simulink model "Model16"  (R2016a)
settings: Solver=FixedStepAuto  StartTime=0  StopTime=inf  FixedStep=0.1  RelTol=1e-3
model workspace (MAT data in the model file):
  c1input = 17
  c2input = 1
  u = 2.9338
settings Model: Creator=CAMILO ANDRES  LastModifiedBy=Luis de la Torre
settings DataIOCC: LimitDataPoints=on  SaveFormat=Array  SaveOutput=off  SignalLogging=off  DSMLogging=off  SaveTime=off
settings DebuggingCC: UnderspecifiedInitializationDetection=Classic  MergeDetectMultiDrivingBlocksExec=none  SolverPrmCheckMsg=warning  FcnCallInpInsideContextMsg=EnableAllAsWarning  StateNameClashWarn=warning
settings HardwareCC: ProdBitPerPointer=32  ProdLargestAtomicFloat=None  ProdIntDivRoundTo=Undefined  ProdEndianess=Unspecified  ProdWordSize=32  ProdHWDeviceType=32-bit Generic
settings ModelReferenceCC: PropagateSignalLabelsOutOfModel=off

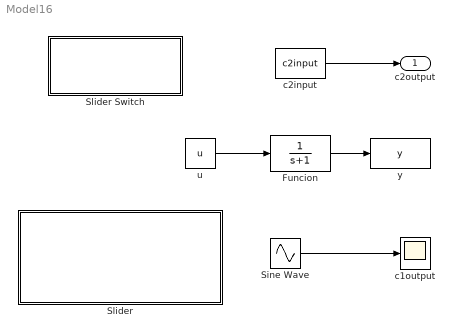
== system Model16 ==
  Funcion : TransferFcn  Denominator=[1 1]  ContinuousStateAttributes='Funcion'
  Sine Wave : Sin  Amplitude=c1input  SampleTime=0
  Slider : Subsystem  DialogController=hmiCreateDDGDialog  IsWebBlock=on  mask(MWDashboardBlock){webBlockId=1239df95-ecf1-4c22-9d9b-c8ac99087a0a, webBlockType=slider, ShowInLibBrowser=on, ShowInitialText=on, HMISrcModelName=Model16}
      mask prompts: webBlockId "WebBlock Id"; webBlockType "WebBlock Type"; HMISrcModelName "Source Model"
      mask help: Set value to tune parameters or variables.
      mask Help: helpview([docroot '/mapfiles/simulink.map'], 'hmi_slider')
      mask Display:
      | if strcmp(get_param(bdroot(gcb),'BlockDiagramType'),'library')
      |  image([(matlabroot) '/toolbox/simulink/hmi/icons/Slider.png'])
      | end
  Slider Switch : Subsystem  DialogController=hmiCreateDDGDialog  IsWebBlock=on  mask(MWDashboardBlock){webBlockId=643e6c24-fc9d-4e9b-8cf7-16ee57daf55e, webBlockType=sliderswitch, ShowInLibBrowser=on, ShowInitialText=on, HMISrcModelName=Model16}
      mask prompts: webBlockId "WebBlock Id"; webBlockType "WebBlock Type"; HMISrcModelName "Source Model"
      mask help: Set on/off value to tune parameters or variables.
      mask Help: helpview([docroot '/mapfiles/simulink.map'], 'hmi_switch')
      mask Display:
      | if strcmp(get_param(bdroot(gcb),'BlockDiagramType'),'library')
      |  image([(matlabroot) '/toolbox/simulink/hmi/icons/SliderSwitch.png'])
      | end
  c1output : Scope
  c2input : Constant  Value=c2input
  u : Constant  Value=u
  y : ToWorkspace  VariableName=y  SampleTime=-1
      settings: MaxDataPoints=1
  c2output : Outport
  wires:
  u/1 -> Funcion/1
  Sine Wave/1 -> c1output/1
  Funcion/1 -> y/1
  c2input/1 -> c2output/1

== system Model16/Slider ==

== system Model16/Slider Switch ==
